simulink model "VCU_PwrMgnt"  (R2023b)
settings: Solver=FixedStepAuto  StartTime=0.0  StopTime=10.0  FixedStep=0.01  RelTol=1e-3
undefined symbols (not defined in the file or in its folder): DiscIntNeverNeededParam
libraries: simulink x45
settings Model: Creator=Administrator  LastModifiedBy=Administrator
settings OptimizationCC: DefaultParameterBehavior=Inlined  EnhancedBackFolding=on  PassReuseOutputArgsAs=Individual arguments  ZeroExternalMemoryAtStartup=off  ZeroInternalMemoryAtStartup=off  OptimizeBlockOrder=speed  DifferentSizesBufferReuse=on  OptimizationCustomize=off  EfficientTunableParamExpr=on
settings DebuggingCC: ParameterTunabilityLossMsg=error
settings HardwareCC: ProdBitPerPointer=32  ProdBitPerSizeT=32  ProdBitPerPtrDiffT=32  ProdLargestAtomicInteger=Long  ProdLargestAtomicFloat=Double  ProdWordSize=32  ProdHWDeviceType=ARM Compatible->ARM Cortex-M
settings SFSimCC: MATLABDynamicMemAlloc=off
settings RTWCC: Description=Embedded Coder  SystemTargetFile=ert.tlc  GenCodeOnly=on  TemplateMakefile=ert_default_tmf  GenerateReport=on  IncludeHyperlinkInReport=on  LaunchReport=on  GenerateTraceInfo=on  GenerateTraceReport=on  GenerateCodeReplacementReport=on
settings CodeAppCC: ForceParamTrailComments=on  IgnoreCustomStorageClasses=off  OperatorAnnotations=on  SimulinkDataObjDesc=on  SFDataObjDesc=on  InsertBlockDesc=on
settings ERTTargetCC: TargetLangStandard=C99 (ISO)  GenerateSampleERTMain=on  InlinedParameterPlacement=NonHierarchical  ERTCustomFileTemplate=example_file_process.tlc

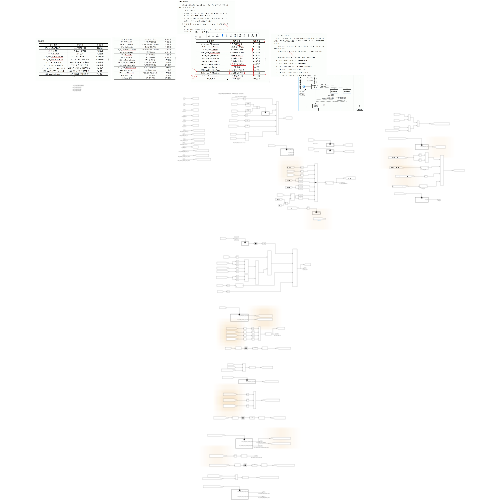
[thumbnail: Simulink's stored preview of the top-level diagram]
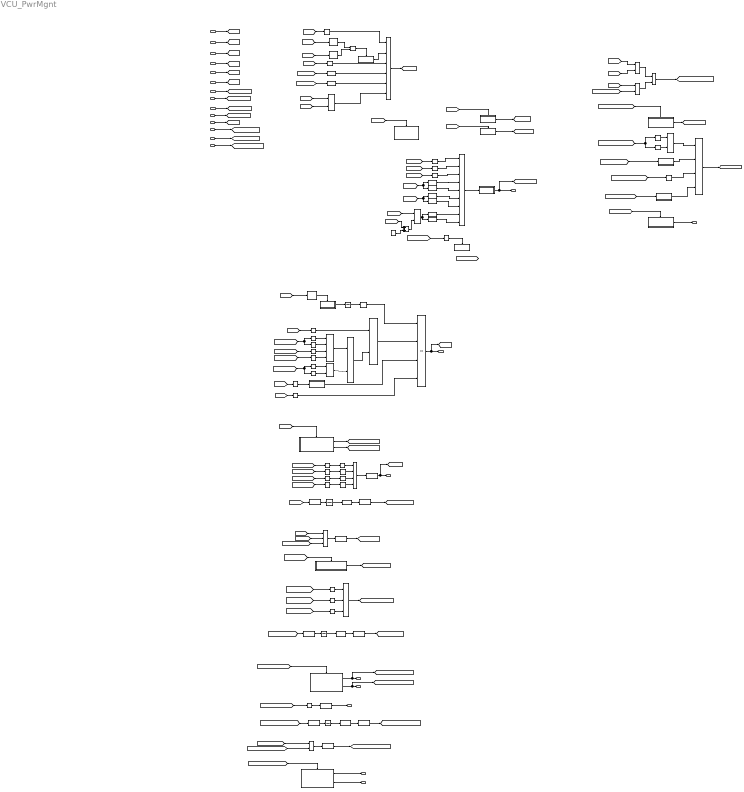
== system VCU_PwrMgnt ==
  note: 钥匙和充电插枪信号至少有一个为1
  note: IGN = 钥匙打到ON档（隐藏条件）
  note: 钥匙上电时间
  note: 钥匙从ON打到START档时，ON档状态是一直保持的
  note: 1.上高压条件判断；
      | 2.上高压过程；
      | 3.上高压完成；
      | 4.上高压失败
  note: 充电上电时间
  ign : Inport
  start : Inport  Port=2
  charge_in : Inport  Port=3
  veh_fault_lev3 : Inport  Port=4
  hv_bat_vol : Inport  Port=5
  hv_mcu_vol : Inport  Port=6
  BMS_SEND_SLOW_ST : Inport  Port=7
  BMS_SEND_FAST_ST : Inport  Port=8
  BMS_SEND_CC_ST : Inport  Port=9
  BMS_SEND_CP_ST : Inport  Port=10
  veh_fault_lev4 : Inport  Port=11
  BMS_SEND_CGE_END_ST : Inport  Port=12
  BMS_SEND_HEART_CNT_10MS : Inport  Port=13
  MCU_SEND_HEART_CNT_10MS1 : Inport  Port=14
  Abs{,1..3} (4 alike) : Abs  SaturateOnIntegerOverflow=off
  Add : Sum
  Compare To Constant{,2..3,13,15,19,22..23} (8 alike) : simulink/Logic and Bit Operations/Compare To Constant  relop===  const=1  OutDataTypeStr=boolean
  Compare To Constant{1,6,29..31} (5 alike) : simulink/Logic and Bit Operations/Compare To Constant  relop===  const=0  OutDataTypeStr=boolean
  Compare To Constant10 : simulink/Logic and Bit Operations/Compare To Constant  relop=<=  const=400  OutDataTypeStr=boolean
  Compare To Constant11 : simulink/Logic and Bit Operations/Compare To Constant  relop=<=  const=1  OutDataTypeStr=boolean
  Compare To Constant12 : simulink/Logic and Bit Operations/Compare To Constant  relop=>=  const=0.9  OutDataTypeStr=boolean
  Compare To Constant14 : simulink/Logic and Bit Operations/Compare To Constant  relop=>=  const=500  OutDataTypeStr=boolean
  Compare To Constant16 : simulink/Logic and Bit Operations/Compare To Constant  relop=>=  const=1  OutDataTypeStr=boolean
  Compare To Constant{17,21,24..27} (6 alike) : simulink/Logic and Bit Operations/Compare To Constant  relop=<=  const=3.0  OutDataTypeStr=boolean
  Compare To Constant18 : simulink/Logic and Bit Operations/Compare To Constant  relop===  const=7  OutDataTypeStr=boolean
  Compare To Constant20 : simulink/Logic and Bit Operations/Compare To Constant  relop=>=  const=1  OutDataTypeStr=boolean
  Compare To Constant28 : simulink/Logic and Bit Operations/Compare To Constant  relop=<=  const=6000  OutDataTypeStr=boolean
  Compare To Constant32 : simulink/Logic and Bit Operations/Compare To Constant  relop=>=  const=200  OutDataTypeStr=boolean
  Compare To Constant33 : simulink/Logic and Bit Operations/Compare To Constant  relop===  const=3  OutDataTypeStr=boolean
  Compare To Constant34 : simulink/Logic and Bit Operations/Compare To Constant  relop=>  const=300  OutDataTypeStr=boolean
  Compare To Constant35 : simulink/Logic and Bit Operations/Compare To Constant  relop=<=  const=7  OutDataTypeStr=boolean
  Compare To Constant36 : simulink/Logic and Bit Operations/Compare To Constant  relop=>=  const=1  OutDataTypeStr=boolean
  Compare To Constant37 : simulink/Logic and Bit Operations/Compare To Constant  relop===  const=2  OutDataTypeStr=boolean
  Compare To Constant4 : simulink/Logic and Bit Operations/Compare To Constant  relop=<=  const=500  OutDataTypeStr=boolean
  Compare To Constant5 : simulink/Logic and Bit Operations/Compare To Constant  relop=<=  const=500  OutDataTypeStr=boolean
  Compare To Constant7 : simulink/Logic and Bit Operations/Compare To Constant  relop=>=  const=320  OutDataTypeStr=boolean
  Compare To Constant8 : simulink/Logic and Bit Operations/Compare To Constant  relop=<=  const=400  OutDataTypeStr=boolean
  Compare To Constant9 : simulink/Logic and Bit Operations/Compare To Constant  relop=>=  const=320  OutDataTypeStr=boolean
  Constant : Constant  Value=0.01
  Data Type Conversion{,1..9} (10 alike) : DataTypeConversion  SaturateOnIntegerOverflow=off  RndMeth=Floor
  Detect Rise Nonnegative : simulink/Logic and Bit Operations/Detect Rise Nonnegative  vinit=0  OutDataTypeStr=boolean
  Detect Rise Nonnegative1 : simulink/Logic and Bit Operations/Detect Rise Nonnegative  vinit=0  OutDataTypeStr=boolean
  Detect Rise Nonnegative2 : simulink/Logic and Bit Operations/Detect Rise Nonnegative  vinit=0  OutDataTypeStr=boolean
  Discrete-Time Integrator{,1..3} (4 alike) : DiscreteIntegrator  SampleTime=-1  ICPrevOutput=DiscIntNeverNeededParam  ICPrevScaledInput=DiscIntNeverNeededParam
  Divide : Product  Inputs=*/  RndMeth=Zero  SaturateOnIntegerOverflow=on
  Enabled Subsystem : Subsystem  TreatAsAtomicUnit=on
  Enabled Subsystem1 : Subsystem  TreatAsAtomicUnit=on
  Enabled Subsystem10 : Subsystem  TreatAsAtomicUnit=on
  Enabled Subsystem2 : Subsystem  TreatAsAtomicUnit=on
  Enabled Subsystem3 : Subsystem  TreatAsAtomicUnit=on
  Enabled Subsystem4 : Subsystem  TreatAsAtomicUnit=on
  Enabled Subsystem5 : Subsystem  TreatAsAtomicUnit=on
  Enabled Subsystem6 : Subsystem  TreatAsAtomicUnit=on
  Enabled Subsystem7 : Subsystem  TreatAsAtomicUnit=on
  Enabled Subsystem8 : Subsystem  TreatAsAtomicUnit=on
  Enabled Subsystem9 : Subsystem  TreatAsAtomicUnit=on
  FILT_NE : Subsystem  mask{FIT_NUM=10}
  FILT_NE1 : Subsystem  mask{FIT_NUM=10}
  Logical Operator{,2,5,12..13,15} (6 alike) : Logic  Operator=OR  AllPortsSameDT=off  OutDataTypeStr=boolean
  Logical Operator1 : Logic  Inputs=6  AllPortsSameDT=off  OutDataTypeStr=boolean
  Logical Operator10 : Logic  Operator=OR  Inputs=3  AllPortsSameDT=off  OutDataTypeStr=boolean
  Logical Operator11 : Logic  Inputs=3  AllPortsSameDT=off  OutDataTypeStr=boolean
  Logical Operator{6..7,14,16} (4 alike) : Logic  AllPortsSameDT=off  OutDataTypeStr=boolean
  Logical Operator17 : Logic  Inputs=4  AllPortsSameDT=off  OutDataTypeStr=boolean
  Logical Operator3 : Logic  Inputs=9  AllPortsSameDT=off  OutDataTypeStr=boolean
  Logical Operator4 : Logic  Inputs=4  AllPortsSameDT=off  OutDataTypeStr=boolean
  Logical Operator8 : Logic  Operator=OR  Inputs=4  AllPortsSameDT=off  OutDataTypeStr=boolean
  Logical Operator9 : Logic  Inputs=4  AllPortsSameDT=off  OutDataTypeStr=boolean
  Subsystem : Subsystem  mask{FIT_NUM=80}
  Subsystem1 : Subsystem  mask{FIT_NUM=3000}
  Triggered Subsystem : Subsystem  TreatAsAtomicUnit=on
  HV_PRE_COMPLETE : Outport
  HV_OFF_EN : Outport  Port=2
  HV_OFF_PRE_OK : Outport  Port=3
  VCU_SEND_MCU_ENABLE : Outport  Port=4
  VCU_SEND_MCU_POWER_DOWN_CMD : Outport  Port=5
  MCU_SEND_ACT_DISCGE_OK : Outport  Port=6
  VCU_SEND_BMS_SLEEP_CMD : Outport  Port=7
  VCU_SEND_MCU_SLEEP_CMD : Outport  Port=8
  ECU_ST : Outport  Port=9
  wires:
  ign/1 -> [ign]
  start/1 -> [start]
  charge_in/1 -> [charge_in]
  veh_fault_lev3/1 -> [veh_fault_lev3]
  [ign] -> Compare To Constant/1
  [start] -> Detect Rise Nonnegative/1
  [charge_in] -> Detect Rise Nonnegative1/1
  Detect Rise Nonnegative/1 -> Logical Operator/1
  Detect Rise Nonnegative1/1 -> Logical Operator/2
  Logical Operator/1 -> Triggered Subsystem/Trigger
  [veh_fault_lev3] -> Compare To Constant1/1
  Compare To Constant/1 -> Logical Operator1/1
  Triggered Subsystem/1(Out1) -> Logical Operator1/2
  Compare To Constant1/1 -> Logical Operator1/3
  [ign] -> Logical Operator2/1
  [charge_in] -> Logical Operator2/2
  Logical Operator1/1 -> [HV_ON_CMD]
  [ign] -> Enabled Subsystem/Enable
  [charge_in] -> Enabled Subsystem1/Enable
  Enabled Subsystem/1(Out1) -> [IGN_ON_TIME]
  Enabled Subsystem1/1(Out1) -> [CHARGE_IN_TIME]
  [IGN_ON_TIME] -> Compare To Constant4/1
  [CHARGE_IN_TIME] -> Compare To Constant5/1
  Compare To Constant4/1 -> Logical Operator1/4
  Compare To Constant5/1 -> Logical Operator1/5
  Logical Operator2/1 -> Logical Operator1/6
  [HV_ON_CMD] -> Enabled Subsystem2/Enable
  hv_bat_vol/1 -> [hv_bat_vol]
  hv_mcu_vol/1 -> [hv_mcu_vol]
  [HV_NEG_RLY] -> Compare To Constant2/1
  [HV_PRE_RLY] -> Compare To Constant3/1
  [HV_POS_RLY] -> Compare To Constant6/1
  [hv_mcu_vol] -> Compare To Constant8/1, Compare To Constant7/1
  [hv_bat_vol] -> Compare To Constant9/1, Compare To Constant10/1
  [hv_mcu_vol] -> Divide/1
  [hv_bat_vol] -> Add/1
  Divide/1 -> Compare To Constant11/1, Compare To Constant12/1
  Compare To Constant12/1 -> Logical Operator3/8
  Compare To Constant6/1 -> Logical Operator3/3
  Compare To Constant7/1 -> Logical Operator3/4
  Compare To Constant3/1 -> Logical Operator3/2
  Compare To Constant2/1 -> Logical Operator3/1
  Compare To Constant8/1 -> Logical Operator3/5
  Compare To Constant9/1 -> Logical Operator3/6
  Compare To Constant11/1 -> Logical Operator3/9
  Compare To Constant10/1 -> Logical Operator3/7
  Constant/1 -> Add/2
  Add/1 -> Divide/2
  Logical Operator3/1 -> Subsystem/1(In1)
  Subsystem/1(Out1) -> [HV_PRE_COMPLETE], HV_PRE_COMPLETE/1
  [HV_PRE_COMPLETE] -> Compare To Constant13/1
  Compare To Constant13/1 -> Enabled Subsystem3/Enable
  [start] -> Detect Rise Nonnegative2/1
  Detect Rise Nonnegative2/1 -> Enabled Subsystem4/Enable
  Enabled Subsystem4/1(Out1) -> Discrete-Time Integrator/1
  Discrete-Time Integrator/1 -> Compare To Constant14/1
  [charge_in] -> Compare To Constant15/1
  BMS_SEND_SLOW_ST/1 -> [BMS_SEND_SLOW_ST]
  BMS_SEND_FAST_ST/1 -> [BMS_SEND_FAST_ST]
  BMS_SEND_CP_ST/1 -> [BMS_SEND_CP_ST]
  BMS_SEND_CC_ST/1 -> [BMS_SEND_CC_ST]
  [BMS_SEND_SLOW_ST] -> Compare To Constant16/1, Compare To Constant17/1
  [BMS_SEND_CP_ST] -> Compare To Constant18/1
  [BMS_SEND_CC_ST] -> Compare To Constant19/1
  Compare To Constant16/1 -> Logical Operator4/1
  Compare To Constant17/1 -> Logical Operator4/2
  Compare To Constant18/1 -> Logical Operator4/3
  Compare To Constant19/1 -> Logical Operator4/4
  Logical Operator4/1 -> Logical Operator5/1
  Compare To Constant21/1 -> Logical Operator6/2
  Compare To Constant20/1 -> Logical Operator6/1
  [BMS_SEND_FAST_ST] -> Compare To Constant21/1, Compare To Constant20/1
  Logical Operator6/1 -> Logical Operator5/2
  Compare To Constant15/1 -> Logical Operator7/1
  Logical Operator5/1 -> Logical Operator7/2
  [veh_fault_lev3] -> Compare To Constant22/1
  Compare To Constant22/1 -> Subsystem1/1(In1)
  veh_fault_lev4/1 -> [veh_fault_lev4]
  [veh_fault_lev4] -> Compare To Constant23/1
  Compare To Constant14/1 -> Logical Operator8/1
  Logical Operator7/1 -> Logical Operator8/2
  Subsystem1/1(Out1) -> Logical Operator8/3
  Compare To Constant23/1 -> Logical Operator8/4
  Logical Operator8/1 -> [HV_OFF_EN], HV_OFF_EN/1
  [HV_OFF_EN] -> Enabled Subsystem5/Enable
  Enabled Subsystem5/1(VCU_SEND_HV_OFF_CMD) -> [VCU_SEND_HV_OFF_CMD]
  Enabled Subsystem5/2(VCU_SEND_MOTOR_OFF_CMD) -> [VCU_SEND_MOTOR_OFF_CMD]
  [MCU_SEND_ACT_TQ] -> Abs/1
  [MCU_SEND_ACT_SPD] -> Abs1/1
  [BMS_SEND_BATCUR] -> Abs2/1
  [VEL_SPD] -> Abs3/1
  Abs3/1 -> Compare To Constant27/1
  Abs2/1 -> Compare To Constant26/1
  Abs1/1 -> Compare To Constant25/1
  Abs/1 -> Compare To Constant24/1
  Compare To Constant25/1 -> Logical Operator9/2
  Compare To Constant24/1 -> Logical Operator9/1
  Compare To Constant26/1 -> Logical Operator9/3
  Compare To Constant27/1 -> Logical Operator9/4
  Logical Operator9/1 -> Data Type Conversion/1
  Data Type Conversion/1 -> [HV_OFF_PRE_OK], HV_OFF_PRE_OK/1
  [HV_OFF_EN] -> Data Type Conversion1/1
  Data Type Conversion1/1 -> Discrete-Time Integrator1/1
  Discrete-Time Integrator1/1 -> Compare To Constant28/1
  Compare To Constant28/1 -> Data Type Conversion2/1
  Data Type Conversion2/1 -> [HV_OFF_PRE_OVER_TIME]
  [veh_fault_lev4] -> Logical Operator10/1
  [HV_OFF_PRE_OVER_TIME] -> Logical Operator10/3
  [HV_OFF_PRE_OK] -> Logical Operator10/2
  Logical Operator10/1 -> Data Type Conversion3/1
  Data Type Conversion3/1 -> [HV_OFF_ACT_START]
  [HV_OFF_ACT_START] -> Enabled Subsystem6/Enable
  Enabled Subsystem6/1(VCU_SEND_HV_OFF_CMD) -> [VCU_SEND_BMS_OFF_CMD]
  [BMS_SEND_POS_RLY] -> Compare To Constant29/1
  [BMS_SEND_NEG_RLY] -> Compare To Constant30/1
  [BMS_SEND_PRG_RLY] -> Compare To Constant31/1
  Compare To Constant29/1 -> Logical Operator11/1
  Compare To Constant30/1 -> Logical Operator11/2
  Compare To Constant31/1 -> Logical Operator11/3
  Logical Operator11/1 -> [VCU_SEND_BMS_HV_OFF_OK]
  Data Type Conversion5/1 -> [HV_OFF_ACT_OVER_TIME]
  Compare To Constant32/1 -> Data Type Conversion5/1
  Discrete-Time Integrator2/1 -> Compare To Constant32/1
  Data Type Conversion4/1 -> Discrete-Time Integrator2/1
  [VCU_SEND_BMS_OFF_CMD] -> Data Type Conversion4/1
  Enabled Subsystem7/1(VCU_SEND_MCU_ENABLE_CMD) -> [VCU_SEND_MCU_ENABLE_CMD], VCU_SEND_MCU_ENABLE/1
  [VCU_SEND_BMS_HV_OFF_OK] -> Enabled Subsystem7/Enable
  Enabled Subsystem7/2(VCU_SEND_MCU_POWER_DOWN_CMD) -> [VCU_SEND_MCU_POWER_DOWN_CMD], VCU_SEND_MCU_POWER_DOWN_CMD/1
  [VCU_SEND_ACT_DISCGE_ST] -> Compare To Constant33/1
  Compare To Constant33/1 -> Data Type Conversion6/1
  Data Type Conversion6/1 -> MCU_SEND_ACT_DISCGE_OK/1
  [VCU_SEND_MCU_POWER_DOWN_CMD] -> Data Type Conversion7/1
  Data Type Conversion7/1 -> Discrete-Time Integrator3/1
  Discrete-Time Integrator3/1 -> Compare To Constant34/1
  Compare To Constant34/1 -> Data Type Conversion8/1
  Data Type Conversion8/1 -> [MCU_SEND_ACT_DISCGE_OVER_TIME]
  [HV_OFF_ACT_OVER_TIME] -> Logical Operator12/1
  [MCU_SEND_ACT_DISCGE_OVER_TIME] -> Logical Operator12/2
  Logical Operator12/1 -> Data Type Conversion9/1
  Data Type Conversion9/1 -> [VCU_SEND_SLEEP_CMD]
  [VCU_SEND_SLEEP_CMD] -> Enabled Subsystem8/Enable
  Enabled Subsystem8/1(VCU_SEND_BMS_SLEEP_CMD) -> VCU_SEND_BMS_SLEEP_CMD/1
  Enabled Subsystem8/2(VCU_SEND_MCU_SLEEP_CMD) -> VCU_SEND_MCU_SLEEP_CMD/1
  BMS_SEND_CGE_END_ST/1 -> [BMS_SEND_CGE_END_ST]
  [ign] -> Logical Operator13/1
  [start] -> Logical Operator13/2
  [charge_in] -> Logical Operator14/1
  [BMS_SEND_CGE_END_ST] -> Logical Operator14/2
  Logical Operator13/1 -> Logical Operator15/1
  Logical Operator14/1 -> Logical Operator15/2
  Logical Operator15/1 -> [VCU_SEND_LV_POWER_ON_CMD]
  [VCU_SEND_LV_POWER_ON_CMD] -> Enabled Subsystem9/Enable
  Enabled Subsystem9/1(VCU_WAKE_RLY_OUT) -> [VCU_WAKE_RLY_OUT]
  [BMS_SEND_BAT_ST] -> Compare To Constant36/1, Compare To Constant35/1
  Compare To Constant35/1 -> Logical Operator16/1
  Compare To Constant36/1 -> Logical Operator16/2
  Logical Operator16/1 -> Logical Operator17/1
  BMS_SEND_HEART_CNT_10MS/1 -> [BMS_SEND_HEAT_CNT_10MS]
  [BMS_SEND_HEAT_CNT_10MS] -> FILT_NE/1(In1)
  [MCU_SEND_MOT_INI_ST] -> Compare To Constant37/1
  MCU_SEND_HEART_CNT_10MS1/1 -> [MCU_SEND_HEAT_CNT_10MS]
  [MCU_SEND_HEAT_CNT_10MS] -> FILT_NE1/1(In1)
  FILT_NE/1(Out1) -> Logical Operator17/2
  Compare To Constant37/1 -> Logical Operator17/3
  FILT_NE1/1(Out1) -> Logical Operator17/4
  Logical Operator17/1 -> [ECU_LV_PWR_OK]
  [ECU_LV_PWR_OK] -> Enabled Subsystem10/Enable
  Enabled Subsystem10/1(ECU_ST) -> ECU_ST/1

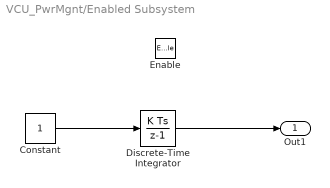
== system VCU_PwrMgnt/Enabled Subsystem ==
  Enable : EnablePort
  Constant : Constant  OutDataTypeStr=single
  Discrete-Time Integrator : DiscreteIntegrator  SampleTime=-1  ICPrevOutput=DiscIntNeverNeededParam  ICPrevScaledInput=DiscIntNeverNeededParam
  Out1 : Outport
  wires:
  Constant/1 -> Discrete-Time Integrator/1
  Discrete-Time Integrator/1 -> Out1/1

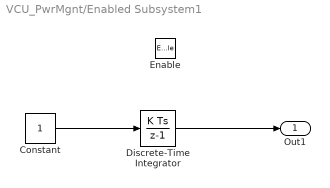
== system VCU_PwrMgnt/Enabled Subsystem1 ==
  Enable : EnablePort
  Constant : Constant  OutDataTypeStr=single
  Discrete-Time Integrator : DiscreteIntegrator  SampleTime=-1  ICPrevOutput=DiscIntNeverNeededParam  ICPrevScaledInput=DiscIntNeverNeededParam
  Out1 : Outport
  wires:
  Discrete-Time Integrator/1 -> Out1/1
  Constant/1 -> Discrete-Time Integrator/1

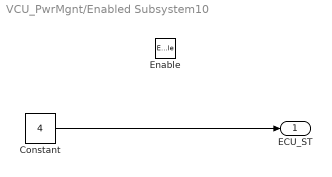
== system VCU_PwrMgnt/Enabled Subsystem10 ==
  Enable : EnablePort
  Constant : Constant  Value=4
  ECU_ST : Outport
  wires:
  Constant/1 -> ECU_ST/1

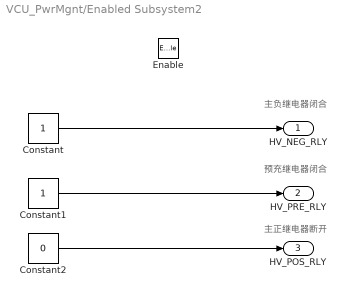
== system VCU_PwrMgnt/Enabled Subsystem2 ==
  note: 主负继电器闭合
  note: 预充继电器闭合
  note: 主正继电器断开
  Enable : EnablePort
  Constant : Constant
  Constant1 : Constant
  Constant2 : Constant  Value=0
  HV_NEG_RLY : Outport
  HV_PRE_RLY : Outport  Port=2
  HV_POS_RLY : Outport  Port=3
  wires:
  Constant/1 -> HV_NEG_RLY/1
  Constant1/1 -> HV_PRE_RLY/1
  Constant2/1 -> HV_POS_RLY/1

== system VCU_PwrMgnt/Enabled Subsystem3 ==
  Enable : EnablePort
  Constant : Constant  OutDataTypeStr=uint8
  HV_POS_RLY : Outport
  wires:
  Constant/1 -> HV_POS_RLY/1

== system VCU_PwrMgnt/Enabled Subsystem4 ==
  Enable : EnablePort
  Constant : Constant
  Out1 : Outport
  wires:
  Constant/1 -> Out1/1

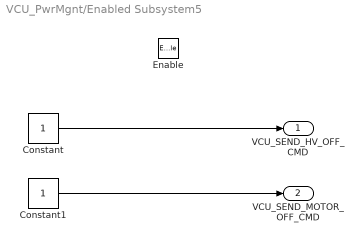
== system VCU_PwrMgnt/Enabled Subsystem5 ==
  Enable : EnablePort
  Constant : Constant  OutDataTypeStr=uint8
  Constant1 : Constant  OutDataTypeStr=uint8
  VCU_SEND_HV_OFF_CMD : Outport
  VCU_SEND_MOTOR_OFF_CMD : Outport  Port=2
  wires:
  Constant/1 -> VCU_SEND_HV_OFF_CMD/1
  Constant1/1 -> VCU_SEND_MOTOR_OFF_CMD/1

== system VCU_PwrMgnt/Enabled Subsystem6 ==
  Enable : EnablePort
  Constant : Constant
  VCU_SEND_HV_OFF_CMD : Outport
  wires:
  Constant/1 -> VCU_SEND_HV_OFF_CMD/1

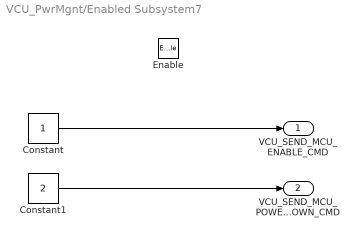
== system VCU_PwrMgnt/Enabled Subsystem7 ==
  Enable : EnablePort
  Constant : Constant
  Constant1 : Constant  Value=2
  VCU_SEND_MCU_ENABLE_CMD : Outport
  VCU_SEND_MCU_POWER_DOWN_CMD : Outport  Port=2
  wires:
  Constant/1 -> VCU_SEND_MCU_ENABLE_CMD/1
  Constant1/1 -> VCU_SEND_MCU_POWER_DOWN_CMD/1

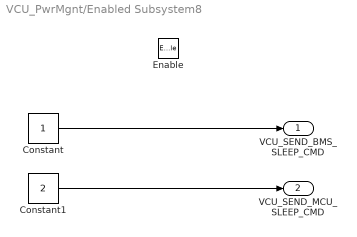
== system VCU_PwrMgnt/Enabled Subsystem8 ==
  Enable : EnablePort
  Constant : Constant
  Constant1 : Constant  Value=2
  VCU_SEND_BMS_SLEEP_CMD : Outport
  VCU_SEND_MCU_SLEEP_CMD : Outport  Port=2
  wires:
  Constant1/1 -> VCU_SEND_MCU_SLEEP_CMD/1
  Constant/1 -> VCU_SEND_BMS_SLEEP_CMD/1

== system VCU_PwrMgnt/Enabled Subsystem9 ==
  Enable : EnablePort
  Constant : Constant
  VCU_WAKE_RLY_OUT : Outport
  wires:
  Constant/1 -> VCU_WAKE_RLY_OUT/1

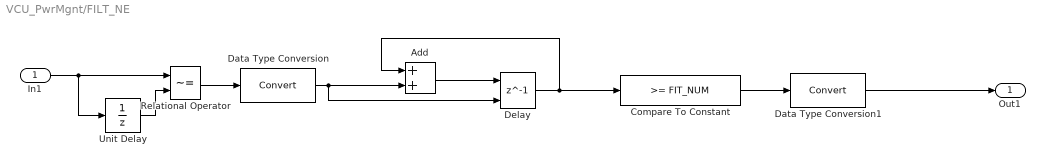
== system VCU_PwrMgnt/FILT_NE ==
  In1 : Inport
  Add : Sum
  Compare To Constant : simulink/Logic and Bit Operations/Compare To Constant  relop=>=  const=FIT_NUM  OutDataTypeStr=boolean
  Data Type Conversion : DataTypeConversion  SaturateOnIntegerOverflow=off  RndMeth=Floor
  Data Type Conversion1 : DataTypeConversion  SaturateOnIntegerOverflow=off  RndMeth=Floor
  Delay : Delay  DelayLength=1  ExternalReset=Falling
      settings: InputPortMap=u0,r5
  Relational Operator : RelationalOperator  Operator=~=  OutDataTypeStr=boolean  RndMeth=Simplest  InputSameDT=off
  Unit Delay : UnitDelay  SampleTime=-1  HasFrameUpgradeWarning=on
  Out1 : Outport
  wires:
  Data Type Conversion1/1 -> Out1/1
  Compare To Constant/1 -> Data Type Conversion1/1
  Delay/1 -> Add/1, Compare To Constant/1
  Add/1 -> Delay/1
  Data Type Conversion/1 -> Add/2, Delay/2
  Relational Operator/1 -> Data Type Conversion/1
  Unit Delay/1 -> Relational Operator/2
  In1/1 -> Relational Operator/1, Unit Delay/1

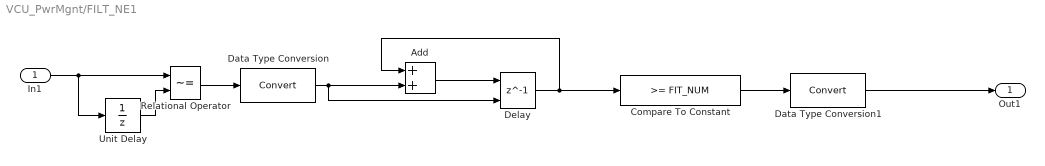
== system VCU_PwrMgnt/FILT_NE1 ==
  In1 : Inport
  Add : Sum
  Compare To Constant : simulink/Logic and Bit Operations/Compare To Constant  relop=>=  const=FIT_NUM  OutDataTypeStr=boolean
  Data Type Conversion : DataTypeConversion  SaturateOnIntegerOverflow=off  RndMeth=Floor
  Data Type Conversion1 : DataTypeConversion  SaturateOnIntegerOverflow=off  RndMeth=Floor
  Delay : Delay  DelayLength=1  ExternalReset=Falling
      settings: InputPortMap=u0,r5
  Relational Operator : RelationalOperator  Operator=~=  OutDataTypeStr=boolean  RndMeth=Simplest  InputSameDT=off
  Unit Delay : UnitDelay  SampleTime=-1  HasFrameUpgradeWarning=on
  Out1 : Outport
  wires:
  In1/1 -> Unit Delay/1, Relational Operator/1
  Unit Delay/1 -> Relational Operator/2
  Relational Operator/1 -> Data Type Conversion/1
  Data Type Conversion/1 -> Delay/2, Add/2
  Add/1 -> Delay/1
  Delay/1 -> Compare To Constant/1, Add/1
  Compare To Constant/1 -> Data Type Conversion1/1
  Data Type Conversion1/1 -> Out1/1

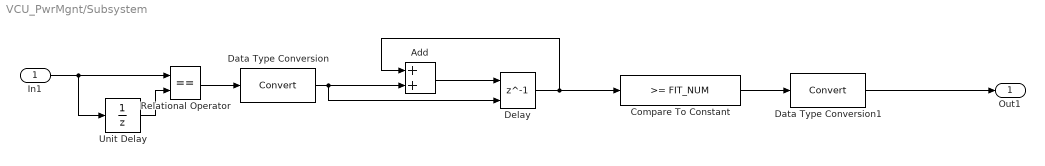
== system VCU_PwrMgnt/Subsystem ==
  In1 : Inport
  Add : Sum
  Compare To Constant : simulink/Logic and Bit Operations/Compare To Constant  relop=>=  const=FIT_NUM  OutDataTypeStr=boolean
  Data Type Conversion : DataTypeConversion  SaturateOnIntegerOverflow=off  RndMeth=Floor
  Data Type Conversion1 : DataTypeConversion  SaturateOnIntegerOverflow=off  RndMeth=Floor
  Delay : Delay  DelayLength=1  ExternalReset=Falling
      settings: InputPortMap=u0,r5
  Relational Operator : RelationalOperator  Operator===  OutDataTypeStr=boolean  RndMeth=Simplest  InputSameDT=off
  Unit Delay : UnitDelay  SampleTime=-1  HasFrameUpgradeWarning=on
  Out1 : Outport
  wires:
  In1/1 -> Unit Delay/1, Relational Operator/1
  Unit Delay/1 -> Relational Operator/2
  Relational Operator/1 -> Data Type Conversion/1
  Data Type Conversion/1 -> Delay/2, Add/2
  Add/1 -> Delay/1
  Delay/1 -> Compare To Constant/1, Add/1
  Compare To Constant/1 -> Data Type Conversion1/1
  Data Type Conversion1/1 -> Out1/1

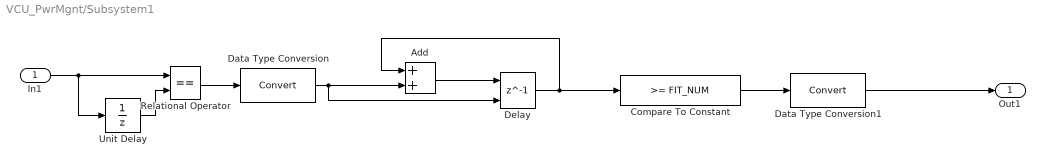
== system VCU_PwrMgnt/Subsystem1 ==
  In1 : Inport
  Add : Sum
  Compare To Constant : simulink/Logic and Bit Operations/Compare To Constant  relop=>=  const=FIT_NUM  OutDataTypeStr=boolean
  Data Type Conversion : DataTypeConversion  SaturateOnIntegerOverflow=off  RndMeth=Floor
  Data Type Conversion1 : DataTypeConversion  SaturateOnIntegerOverflow=off  RndMeth=Floor
  Delay : Delay  DelayLength=1  ExternalReset=Falling
      settings: InputPortMap=u0,r5
  Relational Operator : RelationalOperator  Operator===  OutDataTypeStr=boolean  RndMeth=Simplest  InputSameDT=off
  Unit Delay : UnitDelay  SampleTime=-1  HasFrameUpgradeWarning=on
  Out1 : Outport
  wires:
  Data Type Conversion1/1 -> Out1/1
  Compare To Constant/1 -> Data Type Conversion1/1
  Delay/1 -> Add/1, Compare To Constant/1
  Add/1 -> Delay/1
  Data Type Conversion/1 -> Add/2, Delay/2
  Relational Operator/1 -> Data Type Conversion/1
  Unit Delay/1 -> Relational Operator/2
  In1/1 -> Relational Operator/1, Unit Delay/1

== system VCU_PwrMgnt/Triggered Subsystem ==
  Trigger : TriggerPort  VariantControl=(inherit)
  Constant : Constant
  Out1 : Outport
  wires:
  Constant/1 -> Out1/1
